simulink model "Controller"  (R2024b)
settings: Solver=FixedStepAuto  StartTime=0  StopTime=Tend  FixedStep=Tsim  RelTol=1e-3
values from neighbouring files (symbols this model uses):
  id_cmd = 0    [setup.m]
  id_end = 0.025    [setup.m]    (also in setup_actuator_2026.m; setup_ismb_19.m)
  id_start = 0    [setup.m]    (also in setup_actuator_2026.m; setup_ismb_19.m)
  Ke = 0.003    [setup.m]
  Kf = 1.8    [setup.m]
  Ki_s = R*wb    (= 942.477796077)    [setup.m]    (also in setup_actuator_2026.m = 1413.71669412; setup_ismb_19.m)
  Ki_t = R*wb    (= 942.477796077)    [setup.m]    (also in setup_actuator_2026.m = 1413.71669412; setup_ismb_19.m)
  Kis = -1    [setup.m]    (also in setup_actuator_2026.m; setup_ismb_19.m)
  Kp_s = Ls*wb    (= 1.41371669412)    [setup.m]    (also in setup_actuator_2026.m = 1.05411833699; setup_ismb_19.m)
  Kp_t = Lt*wb    (= 0.942477796077)    [setup.m]    (also in setup_actuator_2026.m = 1.22353633686; setup_ismb_19.m)
  Kt = 0.02    [setup.m]
  Ls = L_alpha_beta(3,3)    [setup.m]    (also in setup_actuator_2026.m; setup_ismb_19.m)
  Lt = L_alpha_beta(1,1)    [setup.m]    (also in setup_actuator_2026.m; setup_ismb_19.m)
  p = 4    [setup.m]    (also in setup_actuator_2026.m = 7; setup_ismb_19.m)
settings Model: Creator=chiba  LastModifiedBy=mhmok
settings SolverCC: AllowMultiTaskInputOutput=on
settings DataIOCC: SaveOutput=off  SaveTime=off
settings OptimizationCC: DefaultParameterBehavior=Inlined  ReuseModelBlockBuffer=off  EnhancedBackFolding=on  PassReuseOutputArgsAs=Individual arguments  ZeroExternalMemoryAtStartup=off  ZeroInternalMemoryAtStartup=off  OptimizeBlockOrder=speed  DifferentSizesBufferReuse=on  EfficientTunableParamExpr=on
settings DebuggingCC: ParameterTunabilityLossMsg=error
settings SFSimCC: MATLABDynamicMemAlloc=off
settings RTWCC: Description=Embedded Coder  SystemTargetFile=ert.tlc  TemplateMakefile=ert_default_tmf  GPUComputeCapability=3.5
settings CodeAppCC: ForceParamTrailComments=on  IgnoreCustomStorageClasses=off  OperatorAnnotations=on  SimulinkDataObjDesc=on  SFDataObjDesc=on  InsertBlockDesc=on
settings ERTTargetCC: TargetLangStandard=C99 (ISO)  ERTCustomFileTemplate=example_file_process.tlc  DynamicArrayContainerType=coder::array

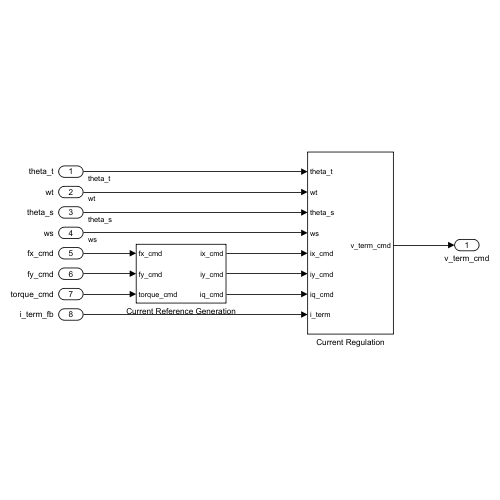
[thumbnail: Simulink's stored preview of the top-level diagram]
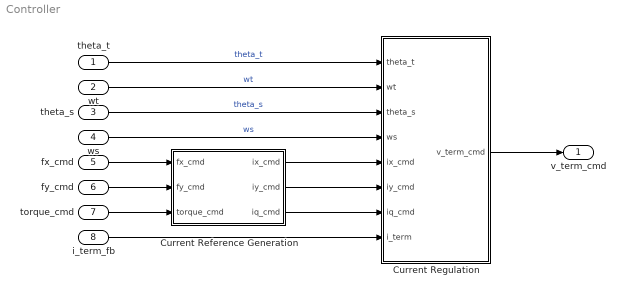
== system Controller ==
  theta_t : Inport  OutDataTypeStr=double  PortDimensions=1  SampleTime=0
  wt : Inport  Port=2  OutDataTypeStr=double  PortDimensions=1
  theta_s : Inport  Port=3  OutDataTypeStr=double  PortDimensions=1  SampleTime=0
  ws : Inport  Port=4  OutDataTypeStr=double  PortDimensions=1
  fx_cmd : Inport  Port=5  OutDataTypeStr=double  PortDimensions=1  SampleTime=0
  fy_cmd : Inport  Port=6  OutDataTypeStr=double  PortDimensions=1  SampleTime=0
  torque_cmd : Inport  Port=7  OutDataTypeStr=double  PortDimensions=1  SampleTime=0
  i_term_fb : Inport  Port=8  OutDataTypeStr=double  PortDimensions=6  SampleTime=0
  Current Reference Generation : Subsystem
  Current Regulation : Subsystem
  v_term_cmd : Outport  OutDataTypeStr=double  PortDimensions=[6 1]  SampleTime=0
  wires:
  Current Reference Generation/3(iq_cmd) -> Current Regulation/7(iq_cmd)
  fy_cmd/1 -> Current Reference Generation/2(fy_cmd)
  torque_cmd/1 -> Current Reference Generation/3(torque_cmd)
  fx_cmd/1 -> Current Reference Generation/1(fx_cmd)
  Current Reference Generation/2(iy_cmd) -> Current Regulation/6(iy_cmd)
  theta_t/1 -> Current Regulation/1(theta_t)  "theta_t"
  i_term_fb/1 -> Current Regulation/8(i_term)
  Current Regulation/1(v_term_cmd) -> v_term_cmd/1
  Current Reference Generation/1(ix_cmd) -> Current Regulation/5(ix_cmd)
  theta_s/1 -> Current Regulation/3(theta_s)  "theta_s"
  ws/1 -> Current Regulation/4(ws)  "ws"
  wt/1 -> Current Regulation/2(wt)  "wt"

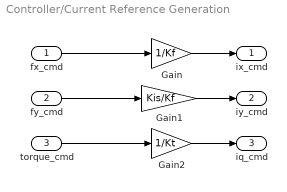
== system Controller/Current Reference Generation ==
  fx_cmd : Inport
  fy_cmd : Inport  Port=2
  torque_cmd : Inport  Port=3
  Gain : Gain  Gain=1/Kf
  Gain1 : Gain  Gain=Kis/Kf
  Gain2 : Gain  Gain=1/Kt
  ix_cmd : Outport
  iy_cmd : Outport  Port=2
  iq_cmd : Outport  Port=3
  wires:
  Gain/1 -> ix_cmd/1
  torque_cmd/1 -> Gain2/1
  fy_cmd/1 -> Gain1/1
  Gain1/1 -> iy_cmd/1
  Gain2/1 -> iq_cmd/1
  fx_cmd/1 -> Gain/1

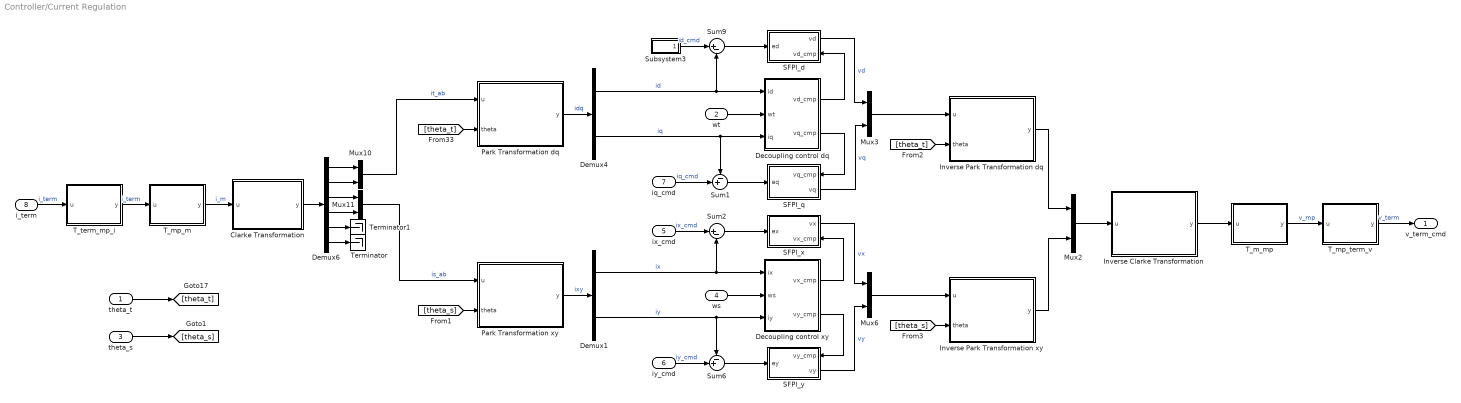
== system Controller/Current Regulation ==
  theta_t : Inport
  wt : Inport  Port=2
  theta_s : Inport  Port=3
  ws : Inport  Port=4
  ix_cmd : Inport  Port=5
  iy_cmd : Inport  Port=6
  iq_cmd : Inport  Port=7
  i_term : Inport  Port=8
  Clarke Transformation : MATLAB Function  TreatAsAtomicUnit=on
  Decoupling control dq : Subsystem
  Decoupling control xy : Subsystem
  Demux1 : Demux  Outputs=2
  Demux4 : Demux  Outputs=2
  Demux6 : Demux  Outputs=6
  Inverse Clarke Transformation : MATLAB Function  TreatAsAtomicUnit=on
  Inverse Park Transformation dq : MATLAB Function  TreatAsAtomicUnit=on
  Inverse Park Transformation xy : MATLAB Function  TreatAsAtomicUnit=on
  Mux{2..3,6,10..11} (5 alike) : Mux  Inputs=2
  Park Transformation dq : MATLAB Function  TreatAsAtomicUnit=on
  Park Transformation xy : MATLAB Function  TreatAsAtomicUnit=on
  SFPI_d : Subsystem
      settings: PortSchema="{\"entries\":[{\"content\":{\"sides\":[{\"content\":{\"connectorIds\":[\"In1\"]},\"type\":\"ConnectorPlacement.EquallySpacedRectSide\",\"uuid\":\"0c9b1a56-be5b-4008-a4be-2c96991c93df\"},{\"content\":{\"connectorIds\":[\"Out1\",\"In2\"],\"side\":\"RIGHT\"},\"type\":\"ConnectorPlacement.EquallySpacedRectSide\",\"uuid\":\"62f10227-e6d2-436b-83cf-88635ef632ae\"},{\"content\":{\"side\":\"TOP\"},\"type\":\"ConnectorPlacement.EquallySpacedRectSide\",\"uuid\":\"775f088e-b169-44e0-8f62-950b5ccb7049\"}]},\"type\":\"ConnectorPlacement.EquallySpacedConnector\",\"uuid\":\"a91bb4f4-db64-42d6-b57d-9e899cd3ff7e\"}],\"packageUris\":[\"http://schema.mathworks.com/mf0/Connector/R2020b\"],\"version\":\"1.0\"}"
  SFPI_q : Subsystem
      settings: PortSchema="{\"entries\":[{\"content\":{\"sides\":[{\"content\":{\"connectorIds\":[\"In1\"]},\"type\":\"ConnectorPlacement.EquallySpacedRectSide\",\"uuid\":\"0c9b1a56-be5b-4008-a4be-2c96991c93df\"},{\"content\":{\"connectorIds\":[\"In2\",\"Out1\"],\"side\":\"RIGHT\"},\"type\":\"ConnectorPlacement.EquallySpacedRectSide\",\"uuid\":\"62f10227-e6d2-436b-83cf-88635ef632ae\"},{\"content\":{\"side\":\"TOP\"},\"type\":\"ConnectorPlacement.EquallySpacedRectSide\",\"uuid\":\"775f088e-b169-44e0-8f62-950b5ccb7049\"}]},\"type\":\"ConnectorPlacement.EquallySpacedConnector\",\"uuid\":\"a91bb4f4-db64-42d6-b57d-9e899cd3ff7e\"}],\"packageUris\":[\"http://schema.mathworks.com/mf0/Connector/R2020b\"],\"version\":\"1.0\"}"
  SFPI_x : Subsystem
      settings: PortSchema="{\"entries\":[{\"content\":{\"sides\":[{\"content\":{\"connectorIds\":[\"In1\"]},\"type\":\"ConnectorPlacement.EquallySpacedRectSide\",\"uuid\":\"0c9b1a56-be5b-4008-a4be-2c96991c93df\"},{\"content\":{\"connectorIds\":[\"Out1\",\"In2\"],\"side\":\"RIGHT\"},\"type\":\"ConnectorPlacement.EquallySpacedRectSide\",\"uuid\":\"62f10227-e6d2-436b-83cf-88635ef632ae\"},{\"content\":{\"side\":\"TOP\"},\"type\":\"ConnectorPlacement.EquallySpacedRectSide\",\"uuid\":\"775f088e-b169-44e0-8f62-950b5ccb7049\"}]},\"type\":\"ConnectorPlacement.EquallySpacedConnector\",\"uuid\":\"a91bb4f4-db64-42d6-b57d-9e899cd3ff7e\"}],\"packageUris\":[\"http://schema.mathworks.com/mf0/Connector/R2020b\"],\"version\":\"1.0\"}"
  SFPI_y : Subsystem
      settings: PortSchema="{\"entries\":[{\"content\":{\"sides\":[{\"content\":{\"connectorIds\":[\"In1\"]},\"type\":\"ConnectorPlacement.EquallySpacedRectSide\",\"uuid\":\"0c9b1a56-be5b-4008-a4be-2c96991c93df\"},{\"content\":{\"connectorIds\":[\"In2\",\"Out1\"],\"side\":\"RIGHT\"},\"type\":\"ConnectorPlacement.EquallySpacedRectSide\",\"uuid\":\"62f10227-e6d2-436b-83cf-88635ef632ae\"},{\"content\":{\"side\":\"TOP\"},\"type\":\"ConnectorPlacement.EquallySpacedRectSide\",\"uuid\":\"775f088e-b169-44e0-8f62-950b5ccb7049\"}]},\"type\":\"ConnectorPlacement.EquallySpacedConnector\",\"uuid\":\"a91bb4f4-db64-42d6-b57d-9e899cd3ff7e\"}],\"packageUris\":[\"http://schema.mathworks.com/mf0/Connector/R2020b\"],\"version\":\"1.0\"}"
  Subsystem3 : Subsystem
  Sum1 : Sum  Inputs=-+|
  Sum2 : Sum  Inputs=|+-
  Sum6 : Sum  Inputs=-+|
  Sum9 : Sum  Inputs=|+-
  T_m_mp : MATLAB Function  TreatAsAtomicUnit=on
  T_mp_m : MATLAB Function  TreatAsAtomicUnit=on
  T_mp_term_v : MATLAB Function  TreatAsAtomicUnit=on
  T_term_mp_i : MATLAB Function  TreatAsAtomicUnit=on
  Terminator : Terminator
  Terminator1 : Terminator
  v_term_cmd : Outport
  wires:
  theta_s/1 -> [theta_s]
  theta_t/1 -> [theta_t]
  [theta_s] -> Inverse Park Transformation xy/2(theta)
  [theta_t] -> Inverse Park Transformation dq/2(theta)
  iy_cmd/1 -> Sum6/2  "iy_cmd"
  [theta_t] -> Park Transformation dq/2(theta)
  wt/1 -> Decoupling control dq/2(wt)
  Clarke Transformation/1(y) -> Demux6/1
  Sum1/1 -> SFPI_q/1(eq)
  Demux6/2 -> Mux10/2
  Mux10/1 -> Park Transformation dq/1(u)  "it_ab"
  SFPI_d/1(vd) -> Mux3/1  "vd"
  Park Transformation xy/1(y) -> Demux1/1  "ixy"
  Subsystem3/1(id_cmd) -> Sum9/1  "id_cmd"
  [theta_s] -> Park Transformation xy/2(theta)
  Inverse Park Transformation xy/1(y) -> Mux2/2
  Demux6/6 -> Terminator/1
  Sum2/1 -> SFPI_x/1(ex)
  iq_cmd/1 -> Sum1/2  "iq_cmd"
  Inverse Park Transformation dq/1(y) -> Mux2/1
  Sum9/1 -> SFPI_d/1(ed)
  Demux4/2 -> Decoupling control dq/3(iq), Sum1/1  "iq"
  Demux6/5 -> Terminator1/1
  ix_cmd/1 -> Sum2/1  "ix_cmd"
  SFPI_q/1(vq) -> Mux3/2  "vq"
  SFPI_x/1(vx) -> Mux6/1  "vx"
  Demux1/1 -> Decoupling control xy/1(ix), Sum2/2  "ix"
  i_term/1 -> T_term_mp_i/1(u)  "i_term"
  Decoupling control xy/2(vy_cmp) -> SFPI_y/2(vy_cmp)
  Demux4/1 -> Decoupling control dq/1(id), Sum9/2  "id"
  Demux6/4 -> Mux11/2
  Sum6/1 -> SFPI_y/1(ey)
  Demux6/3 -> Mux11/1
  Mux11/1 -> Park Transformation xy/1(u)  "is_ab"
  Mux2/1 -> Inverse Clarke Transformation/1(u)
  Demux1/2 -> Decoupling control xy/3(iy), Sum6/1  "iy"
  Decoupling control xy/1(vx_cmp) -> SFPI_x/2(vx_cmp)
  Decoupling control dq/2(vq_cmp) -> SFPI_q/2(vq_cmp)
  SFPI_y/1(vy) -> Mux6/2  "vy"
  ws/1 -> Decoupling control xy/2(ws)
  Decoupling control dq/1(vd_cmp) -> SFPI_d/2(vd_cmp)
  Demux6/1 -> Mux10/1
  Park Transformation dq/1(y) -> Demux4/1  "idq"
  Mux3/1 -> Inverse Park Transformation dq/1(u)
  Mux6/1 -> Inverse Park Transformation xy/1(u)
  T_term_mp_i/1(y) -> T_mp_m/1(u)  "i_term"
  T_mp_m/1(y) -> Clarke Transformation/1(u)  "i_m"
  Inverse Clarke Transformation/1(y) -> T_m_mp/1(u)
  T_m_mp/1(y) -> T_mp_term_v/1(u)  "v_mp"
  T_mp_term_v/1(y) -> v_term_cmd/1  "v_term"

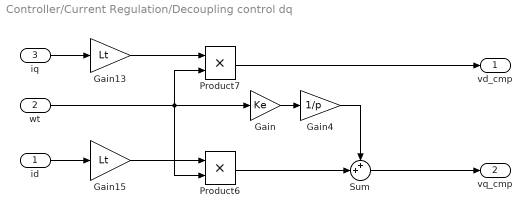
== system Controller/Current Regulation/Decoupling control dq ==
  id : Inport
  wt : Inport  Port=2
  iq : Inport  Port=3
  Gain : Gain  Gain=Ke
  Gain13 : Gain  Gain=Lt
  Gain15 : Gain  Gain=Lt
  Gain4 : Gain  Gain=1/p
  Product6 : Product
  Product7 : Product
  Sum : Sum  Inputs=++|
  vd_cmp : Outport
  vq_cmp : Outport  Port=2
  wires:
  Gain4/1 -> Sum/1
  Sum/1 -> vq_cmp/1
  Product6/1 -> Sum/2
  wt/1 -> Product6/2, Product7/2, Gain/1
  Gain/1 -> Gain4/1
  iq/1 -> Gain13/1
  id/1 -> Gain15/1
  Product7/1 -> vd_cmp/1
  Gain13/1 -> Product7/1
  Gain15/1 -> Product6/1

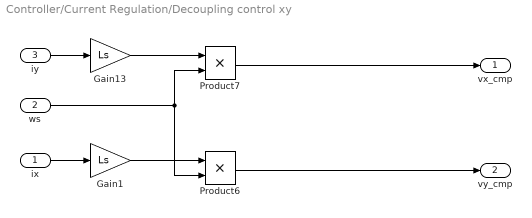
== system Controller/Current Regulation/Decoupling control xy ==
  ix : Inport
  ws : Inport  Port=2
  iy : Inport  Port=3
  Gain1 : Gain  Gain=Ls
  Gain13 : Gain  Gain=Ls
  Product6 : Product
  Product7 : Product
  vx_cmp : Outport
  vy_cmp : Outport  Port=2
  wires:
  Product6/1 -> vy_cmp/1
  iy/1 -> Gain13/1
  ix/1 -> Gain1/1
  Product7/1 -> vx_cmp/1
  Gain13/1 -> Product7/1
  ws/1 -> Product6/2, Product7/2
  Gain1/1 -> Product6/1

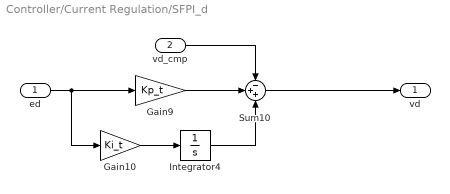
== system Controller/Current Regulation/SFPI_d ==
  ed : Inport
  vd_cmp : Inport  Port=2
  Gain10 : Gain  Gain=Ki_t
  Gain9 : Gain  Gain=Kp_t
  Integrator4 : Integrator
  Sum10 : Sum  Inputs=-++
  vd : Outport
  wires:
  Integrator4/1 -> Sum10/3
  ed/1 -> Gain9/1, Gain10/1
  Sum10/1 -> vd/1
  Gain9/1 -> Sum10/2
  Gain10/1 -> Integrator4/1
  vd_cmp/1 -> Sum10/1

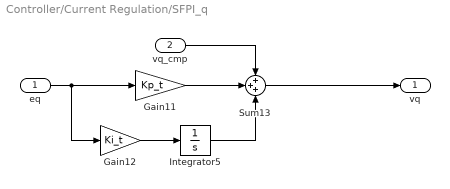
== system Controller/Current Regulation/SFPI_q ==
  eq : Inport
  vq_cmp : Inport  Port=2
  Gain11 : Gain  Gain=Kp_t
  Gain12 : Gain  Gain=Ki_t
  Integrator5 : Integrator
  Sum13 : Sum  Inputs=+++
  vq : Outport
  wires:
  vq_cmp/1 -> Sum13/1
  Gain11/1 -> Sum13/2
  Integrator5/1 -> Sum13/3
  Sum13/1 -> vq/1
  Gain12/1 -> Integrator5/1
  eq/1 -> Gain11/1, Gain12/1

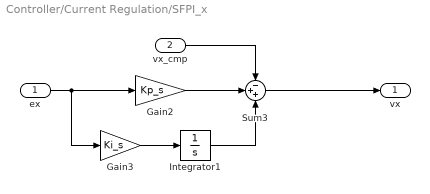
== system Controller/Current Regulation/SFPI_x ==
  ex : Inport
  vx_cmp : Inport  Port=2
  Gain2 : Gain  Gain=Kp_s
  Gain3 : Gain  Gain=Ki_s
  Integrator1 : Integrator
  Sum3 : Sum  Inputs=-++
  vx : Outport
  wires:
  vx_cmp/1 -> Sum3/1
  Sum3/1 -> vx/1
  Integrator1/1 -> Sum3/3
  Gain2/1 -> Sum3/2
  ex/1 -> Gain2/1, Gain3/1
  Gain3/1 -> Integrator1/1

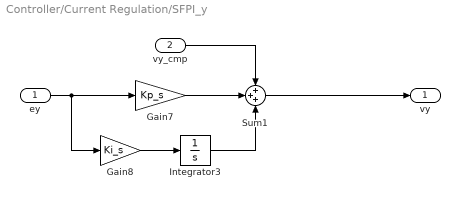
== system Controller/Current Regulation/SFPI_y ==
  ey : Inport
  vy_cmp : Inport  Port=2
  Gain7 : Gain  Gain=Kp_s
  Gain8 : Gain  Gain=Ki_s
  Integrator3 : Integrator
  Sum1 : Sum  Inputs=+++
  vy : Outport
  wires:
  Gain7/1 -> Sum1/2
  Gain8/1 -> Integrator3/1
  ey/1 -> Gain7/1, Gain8/1
  Sum1/1 -> vy/1
  vy_cmp/1 -> Sum1/1
  Integrator3/1 -> Sum1/3

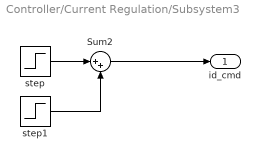
== system Controller/Current Regulation/Subsystem3 ==
  Sum2 : Sum  Inputs=|++
  step : Step  Time=id_start  After=id_cmd  SampleTime=0
  step1 : Step  Time=id_end  After=-id_cmd  SampleTime=0
  id_cmd : Outport
  wires:
  Sum2/1 -> id_cmd/1
  step/1 -> Sum2/1
  step1/1 -> Sum2/2

== matlab function Controller/Current Regulation/Inverse Park Transformation dq ==
  data: u input; y output; theta input
function y  = fcn(u,theta)

y = [cos(theta) -sin(theta); sin(theta) cos(theta)]*u;

== matlab function Controller/Current Regulation/Inverse Park Transformation xy ==
  data: u input; y output; theta input
function y  = fcn(u,theta)

y = [cos(theta) -sin(theta); sin(theta) cos(theta)]*u;

== matlab function Controller/Current Regulation/Park Transformation dq ==
  data: u input; y output; theta input
function y  = fcn(u,theta)

y = [cos(theta) sin(theta); -sin(theta) cos(theta)]*u;

== matlab function Controller/Current Regulation/Park Transformation xy ==
  data: u input; y output; theta input
function y  = fcn(u,theta)

y = [cos(theta) sin(theta); -sin(theta) cos(theta)]*u;

== matlab function Controller/Current Regulation/T_m_mp ==
  data: u input; y output; T_m_mp parameter
function y  = fcn(u, T_m_mp)

y = T_m_mp*u;

== matlab function Controller/Current Regulation/T_term_mp_i ==
  data: u input; y output; T_term_mp_i parameter
function y  = fcn(u, T_term_mp_i)

y = T_term_mp_i*u;

== matlab function Controller/Current Regulation/T_mp_m ==
  data: u input; y output; T_mp_m parameter
function y  = fcn(u, T_mp_m)

y = T_mp_m*u;

== matlab function Controller/Current Regulation/Inverse Clarke Transformation ==
  data: u input; y output; Cr parameter
function y = fcn(u, Cr)

u = [u; 0; 0];

y = Cr\u;

== matlab function Controller/Current Regulation/T_mp_term_v ==
  data: u input; y output; T_mp_term_v parameter
function y  = fcn(u, T_mp_term_v)

y = T_mp_term_v*u;

== matlab function Controller/Current Regulation/Clarke Transformation ==
  data: u input; y output; Cr parameter
function y = fcn(u, Cr)

y = Cr*u;
